simulink model "ICARO3_orientation_controllo_BIPE"  (R2014a)
settings: Solver=FixedStepDiscrete  SolverMode=MultiTasking  StartTime=0.0  StopTime=inf  FixedStep=0.001  RelTol=1e-3
PreLoadFcn:
  | Icaro_path;
  | 
  | load_param;
  | 
  | %override compute_alloc_inside load_param !!!
  | compute_alloc_esa;
  | 
  | load('mag_calib_sim_HIL.mat');
  | 
  | init_adaptive;
InitFcn:
  | %define fast control loop sample time
  | ST = 0.005;
  | 
  | %define filters
  | s = tf('s');
  | 
  | % Derivator (useful in PID controller)
  | D = 0.01*s/(0.01*s+1);
  | 
  | % LP 2nd order filter
  | LP = 42.88/(3.5*s^2 + 19.6*s + 42.88);
  | 
  | %load new DP position controllers
  | progetto_controllo_pos_v1;
undefined symbols (not defined in the file): DiscIntNeverNeededParam, Earth, G, H, INV_PITCH_RANGE, INV_ROLL_RANGE, INV_THROTTLE_RANGE, INV_YAW_RANGE, PITCH_IDX, PITCH_MID, ROLL_IDX, ROLL_MID, RTOL, THROTTLE_DOWN, THROTTLE_IDX, THROTTLE_LOW_THRES, Ts, WGS84, YAW_IDX, YAW_MID
libraries: simulink x15, GPIO_Lib x3, cstblocks x2, aerolibtransform2 x1, STM32_Config_Lib x1
(part 3 of 5)

== system ICARO3_orientation_controllo_BIPE/debug telemtry FLIGHT TEST/GPS ==
  note: lat lon alt_gps gps_status alt_baro_raw
  note: gps: lat, lon, msl_alt, fix_mode + 100*data_valid
  Mux2 : Mux  Inputs=2
  Mux7 : Mux  Inputs=2
  Rate Transition1 : RateTransition  Deterministic=off
  Rate Transition14 : RateTransition  Deterministic=off
  Selector1 : Selector  IndexMode=Zero-based  InputPortWidth=10  Indices=[2]
  Selector2 : Selector  InputPortWidth=2  Indices=2
  Selector3 : Selector  IndexMode=Zero-based  InputPortWidth=10  Indices=[0 1 8]
  Sum : Sum  Inputs=++|
  detect if was 1 in the last 10 samples : Subsystem
  offset : Gain  Gain=100
  GPS : Outport
  wires:
  [TH] -> Selector2/1
  Rate Transition14/1 -> Mux7/2
  [GPS_data] -> Selector3/1, Selector1/1
  Rate Transition1/1 -> Mux7/1
  [GPS_flag] -> detect if was 1 in the last 10 samples/1(In)
  Mux2/1 -> Rate Transition1/1
  Selector3/1 -> Mux2/1
  Selector1/1 -> Sum/2
  Sum/1 -> Mux2/2
  offset/1 -> Sum/1
  Selector2/1 -> Rate Transition14/1
  Mux7/1 -> GPS/1
  detect if was 1 in the last 10 samples/1(Out) -> offset/1

== system ICARO3_orientation_controllo_BIPE/debug telemtry FLIGHT TEST/GPS ECEF ==
  note: CAMBIAMENTI:
      | - Il presente subsystem
      | - wrap_gpsparser
      | - sfun_gpsparser
      | - Latch di ECEF_ref al primo fix GPS
  Demux : Demux  Outputs=[3 3 ]
  Product : Product  Multiplication=Matrix(*)  RndMeth=Zero
  Product1 : Product  Multiplication=Matrix(*)  RndMeth=Zero
  Rate Transition : RateTransition  OutPortSampleTime=1/100
  Rate Transition1 : RateTransition  OutPortSampleTime=1/100
  Sum : Sum  Inputs=-+|
  NED_p : Outport
  NED_v : Outport  Port=2
  wires:
  [ECEF2NED] -> Rate Transition/1
  [ECEF_ref] -> Rate Transition1/1
  Product/1 -> NED_p/1
  Product1/1 -> NED_v/1
  [GPS_data_ECEF] -> Demux/1
  Demux/1 -> Sum/2
  Rate Transition1/1 -> Sum/1
  Sum/1 -> Product/2
  Rate Transition/1 -> Product/1, Product1/1
  Demux/2 -> Product1/2

== system ICARO3_orientation_controllo_BIPE/debug telemtry FLIGHT TEST/MODIFIED Raw IMU data MPU only + RPY AHRS + ALTITUDE (H Hd 0) to be used for AHRS online tuning ==
  ext input : Inport
  Constant : Constant  Value=0  SampleTime=ST
  Manual Switch1 : ManualSwitch  CurrentSetting=0
  Manual Switch2 : ManualSwitch  CurrentSetting=0
  Manual Switch3 : ManualSwitch  CurrentSetting=0
  Mux1 : Mux  Inputs=[3 2 1]
  Mux12 : Mux
  raw imu data : Outport
  wires:
  [MAG_HMC] -> Mux12/4
  Mux1/1 -> Mux12/1
  [RPY_AHRS] -> Mux1/1
  Mux12/1 -> raw imu data/1  "raw_imu_data"
  [H_HD] -> Mux1/2
  Manual Switch3/1 -> Mux12/2
  Manual Switch1/1 -> Mux12/3
  [GYRO_MPU] -> Manual Switch3/2
  [GYRO_ADIS] -> Manual Switch3/1
  [ACC_MPU] -> Manual Switch1/2
  [ACC_ADIS] -> Manual Switch1/1
  Manual Switch2/1 -> Mux1/3
  Constant/1 -> Manual Switch2/1
  ext input/1 -> Manual Switch2/2

== system ICARO3_orientation_controllo_BIPE/debug telemtry FLIGHT TEST/Raw IMU data MPU + HMC + ADC ==
  Mux12 : Mux
  get 1 2 3 4 6 8 : Selector  InputPortWidth=12  Indices=[1 2 3 4 6 8]
  raw imu data : Outport
  wires:
  get 1 2 3 4 6 8/1 -> Mux12/1
  [MAG_HMC] -> Mux12/4
  [ACC_MPU] -> Mux12/3
  [GYRO_MPU] -> Mux12/2
  Mux12/1 -> raw imu data/1  "raw_imu_data"
  [RC_all_channels_usec] -> get 1 2 3 4 6 8/1

== system ICARO3_orientation_controllo_BIPE/debug telemtry FLIGHT TEST/Raw IMU data MPU only + ADC ==
  Mux1 : Mux  Inputs=6
  Mux12 : Mux
  Rate Transition1 : RateTransition  Deterministic=off  OutPortSampleTime=ST
  raw imu data : Outport
  wires:
  Mux12/1 -> raw imu data/1  "raw_imu_data"
  [I_batt] -> Mux1/2
  [V_batt] -> Mux1/1
  [V_batt_filt] -> Mux1/3
  [I_batt_filt] -> Mux1/4
  [P_batt_filt] -> Mux1/5
  [I_consumption_Ah] -> Mux1/6
  Mux1/1 -> Rate Transition1/1
  [GYRO_MPU] -> Mux12/2
  [ACC_MPU] -> Mux12/3
  [MAG_HMC] -> Mux12/4
  Rate Transition1/1 -> Mux12/1

== system ICARO3_orientation_controllo_BIPE/debug telemtry FLIGHT TEST/Raw IMU data packer ==
  Mux12 : Mux  Inputs=5
  raw imu data : Outport
  wires:
  [ACC_MPU] -> Mux12/1
  [GYRO_MPU] -> Mux12/2
  [MAG_HMC] -> Mux12/5
  [GYRO_ITG] -> Mux12/3
  [ACC_ADXL] -> Mux12/4
  Mux12/1 -> raw imu data/1  "raw_imu_data"

== system ICARO3_orientation_controllo_BIPE/debug telemtry FLIGHT TEST/To be used for ADAPT NN online tuning ==
  Mux12 : Mux  Inputs=5
  Selector1 : Selector  InputPortWidth=12  Indices=[7 8 9]
  Selector2 : Selector  InputPortWidth=12  Indices=[10 11 12]
  Selector3 : Selector  InputPortWidth=12  Indices=[1 2 3]
  Selector4 : Selector  InputPortWidth=12  Indices=[4 5 6]
  DEBUG_adapt_contr : Outport
  wires:
  [RPY_AHRS] -> Mux12/1
  Mux12/1 -> DEBUG_adapt_contr/1
  [debug_ADAPT_CONTR] -> Selector2/1, Selector1/1, Selector4/1, Selector3/1
  Selector3/1 -> Mux12/2
  Selector4/1 -> Mux12/3
  Selector1/1 -> Mux12/4
  Selector2/1 -> Mux12/5

== system ICARO3_orientation_controllo_BIPE/debug telemtry FLIGHT TEST/To be used for H PID online tuning ==
  note: hb, zd, 0
  note: y_ref, y, 0
  note: H pid -> D, P, I
  ext input : Inport
  Constant : Constant  Value=0  SampleTime=ST
  Constant1 : Constant  Value=0  SampleTime=ST
  Constant2 : Constant  Value=0  SampleTime=ST
  Manual Switch2 : ManualSwitch  CurrentSetting=0
  Mux1 : Mux  Inputs=[3 2 1]
  Mux12 : Mux
  Mux2 : Mux  Inputs=2
  Mux3 : Mux  Inputs=2
  Selector1 : Selector  InputPortWidth=5  Indices=[1 2 3]
  Selector2 : Selector  InputPortWidth=5  Indices=[4 5]
  raw imu data : Outport
  wires:
  ext input/1 -> Manual Switch2/2
  Constant/1 -> Manual Switch2/1
  Manual Switch2/1 -> Mux1/3
  [H_HD] -> Mux1/2
  Mux12/1 -> raw imu data/1  "raw_imu_data"
  [RPY_AHRS] -> Mux1/1
  Mux1/1 -> Mux12/1
  [debug_H_PID] -> Selector2/1, Selector1/1
  Selector1/1 -> Mux12/2
  Selector2/1 -> Mux3/1
  Constant2/1 -> Mux3/2
  Mux3/1 -> Mux12/3
  [filtInput_debugHPID] -> Mux2/1
  Constant1/1 -> Mux2/2
  Mux2/1 -> Mux12/4

== system ICARO3_orientation_controllo_BIPE/debug telemtry FLIGHT TEST/recupero di mpu9150 data ==
  Mux1 : Mux  Inputs=2
  raw imu data : Outport
  wires:
  Mux1/1 -> raw imu data/1
  [ACC_MPU] -> Mux1/1
  [GYRO_MPU] -> Mux1/2

== system ICARO3_orientation_controllo_BIPE/debug telemtry FLIGHT TEST/test solo RC_all_channel_usec + RSSI + .... ==
  Mux12 : Mux
  Rate Transition1 : RateTransition  Deterministic=off  OutPortSampleTime=ST
  Rate Transition2 : RateTransition  Deterministic=off  OutPortSampleTime=ST
  get 1 2 3 4 6 8 : Selector  InputPortWidth=12  Indices=[1 2 3 4 6 8]
  raw imu data : Outport
  wires:
  get 1 2 3 4 6 8/1 -> Rate Transition1/1
  [RC_all_channels_usec] -> get 1 2 3 4 6 8/1
  Mux12/1 -> raw imu data/1  "raw_imu_data"
  Rate Transition1/1 -> Mux12/1
  [RSSI_VOLT] -> Rate Transition2/1
  [RC_TRPY_refs] -> Mux12/3
  [RC_age] -> Mux12/4
  Rate Transition2/1 -> Mux12/2

== system ICARO3_orientation_controllo_BIPE/debug telemtry FLIGHT TEST1/MODIFIED Raw IMU data MPU only + RPY AHRS + ALTITUDE (H Hd 0) to be used for AHRS online tuning ==
  Mux12 : Mux
  raw imu data : Outport
  wires:
  Mux12/1 -> raw imu data/1  "raw_imu_data"
  [RPY_AHRS_AR] -> Mux12/1
  [ACC_MPU] -> Mux12/2
  [GYRO_MPU] -> Mux12/3
  [H_HD] -> Mux12/4

== system ICARO3_orientation_controllo_BIPE/debug telemtry STATIC TEST/Raw IMU data packer: MPU + MAG_HMC ==
  Manual Switch8 : ManualSwitch  CurrentSetting=0
  Mux12 : Mux  Inputs=3
  raw imu data : Outport
  wires:
  Mux12/1 -> raw imu data/1  "raw_imu_data"
  [GYRO_MPU] -> Mux12/1
  [ACC_MPU] -> Mux12/2
  Manual Switch8/1 -> Mux12/3
  [MAG_MPU] -> Manual Switch8/1
  [MAG_HMC] -> Manual Switch8/2

== system ICARO3_orientation_controllo_BIPE/debug telemtry STATIC TEST/Subsystem ==
  Mux12 : Mux  Inputs=2
  debias_imu_mpu : Outport
  wires:
  [gyro_det_mpu] -> Mux12/2
  Mux12/1 -> debias_imu_mpu/1
  [acc_det_mpu] -> Mux12/1

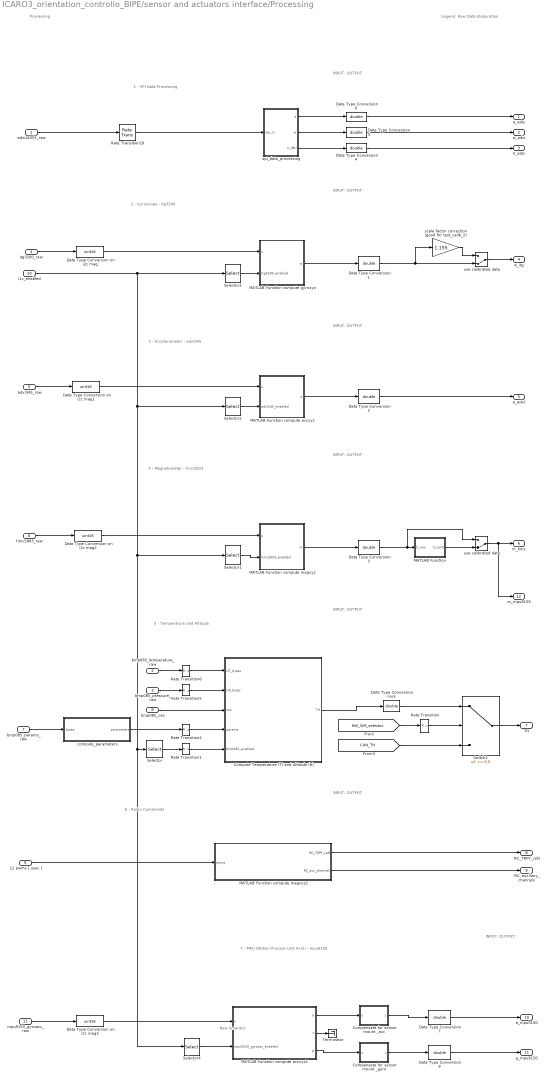
== system ICARO3_orientation_controllo_BIPE/sensor and actuators interface/Processing ==
  note: New Smarabr
  note: Processing
  note: 2 - Gyroscope - itg3200
  note: 1 - SPI Data Processing
  note: 3 - Accelerometer - adxl345
  note: 4 - Magnetometer - hmc5833
  note: 7 - MPU (Motion Process Unit A+G) - mpu9150
  note: 5 - Temperature and Altitude
  note: 6 - Radio Commands
  note: Legend: Raw Data Elaboration
  note: INPUT:
      |
      | OUTPUT:
  note: INPUT:
      |
      | OUTPUT:
  note: INPUT:
      |
      | OUTPUT:
  note: INPUT:
      |
      | OUTPUT:
  note: INPUT:
      |
      | OUTPUT:
  note: INPUT:
      |
      | OUTPUT:
  note: INPUT:
      |
      | OUTPUT:
  adis16355_raw : Inport
  bmp085_temperature_raw : Inport  Port=2
  bmp085_pressure_raw : Inport  Port=3
  itg3200_raw : Inport  Port=4
  adxl345_raw : Inport  Port=5
  hmc5883_raw : Inport  Port=6
  bmp085_params_raw : Inport  Port=7
  bmp085_oss : Inport  Port=8
  12 pwms [ usec ] : Inport  Port=9
  i2c_enabled : Inport  Port=10
  mpu9150_gyroacc_raw : Inport  Port=11
  Compensate for sensor mount _acc : MATLAB Function  TreatAsAtomicUnit=on
  Compensate for sensor mount _gyro : MATLAB Function  TreatAsAtomicUnit=on
  Compute Temperature (T) and Altitude (H) : Subsystem  TreatAsAtomicUnit=on  SystemSampleTime=0.02
  Data Type Conversion mx5 : DataTypeConversion  OutDataTypeStr=double  RndMeth=Round  SaturateOnIntegerOverflow=on
  Data Type Conversion on i2c mag{,1..3} (4 alike) : DataTypeConversion  OutDataTypeStr=uint16
  Data Type Conversion{1..7,9} (8 alike) : DataTypeConversion  OutDataTypeStr=double
  MATLAB Function : MATLAB Function  TreatAsAtomicUnit=on
  MATLAB Function compute accxyz : MATLAB Function  TreatAsAtomicUnit=on
  MATLAB Function compute accxyz1 : MATLAB Function  TreatAsAtomicUnit=on
  MATLAB Function compute gyroxyz : MATLAB Function  TreatAsAtomicUnit=on
  MATLAB Function compute magxyz : MATLAB Function  TreatAsAtomicUnit=on
  MATLAB Function compute magxyz2 : MATLAB Function  TreatAsAtomicUnit=on
  Rate Transition : RateTransition
  Rate Transition{1..2,5..6,18} (5 alike) : RateTransition  Deterministic=off
  Selector : Selector  InputPortWidth=6  Indices=5
  Selector1 : Selector  InputPortWidth=6  Indices=[4]
  Selector2 : Selector  InputPortWidth=6  Indices=3
  Selector3 : Selector  InputPortWidth=6  Indices=[2]
  Selector4 : Selector  InputPortWidth=6  Indices=6
  Switch2 : Switch  Threshold=0.5
  Terminator : Terminator
  compute_parameters : Subsystem
  scale factor correction (good for test_calib_2) : Gain  Gain=1.155
  spi_data_processing : Subsystem
  use calibrated data : ManualSwitch  CurrentSetting=0
  "use calibrated data " : ManualSwitch  CurrentSetting=0
  a_adis : Outport
  w_adis : Outport  Port=2
  V_adis : Outport  Port=3
  w_itg : Outport  Port=4
  a_adxl : Outport  Port=5
  m_hmc : Outport  Port=6
  TH : Outport  Port=7
  RC_TRPY_refs : Outport  Port=8
  RC_auxiliary_channels : Outport  Port=9
  a_mpu9150 : Outport  Port=10
  g_mpu9150 : Outport  Port=11
  m_mpu9150 : Outport  Port=12
  wires:
  Selector4/1 -> MATLAB Function compute accxyz1/2(mpu9150_gyroacc_enabled)
  Data Type Conversion on i2c mag3/1 -> MATLAB Function compute accxyz1/1(u)
  MATLAB Function compute accxyz1/3(g) -> Compensate for sensor mount _gyro/1(u)
  MATLAB Function compute accxyz1/2(t) -> Terminator/1
  Data Type Conversion9/1 -> g_mpu9150/1
  Data Type Conversion7/1 -> a_mpu9150/1
  mpu9150_gyroacc_raw/1 -> Data Type Conversion on i2c mag3/1
  bmp085_temperature_raw/1 -> Rate Transition6/1
  bmp085_pressure_raw/1 -> Rate Transition5/1
  Rate Transition2/1 -> Compute Temperature (T) and Altitude (H)/4(params)
  Rate Transition1/1 -> Compute Temperature (T) and Altitude (H)/5(bmp085_enabled)
  MATLAB Function compute magxyz/1(m) -> Data Type Conversion3/1
  MATLAB Function compute accxyz/1(a) -> Data Type Conversion2/1
  MATLAB Function compute gyroxyz/1(w) -> Data Type Conversion1/1
  Selector/1 -> Rate Transition1/1
  compute_parameters/1(parameters) -> Rate Transition2/1
  Rate Transition/1 -> Switch2/2
  [HW_SIM_selector] -> Rate Transition/1
  [CAN_TH] -> Switch2/3
  Data Type Conversion mx5/1 -> Switch2/1
  Switch2/1 -> TH/1
  scale factor correction (good for test_calib_2)/1 -> "use calibrated data "/1
  "use calibrated data "/1 -> w_itg/1
  use calibrated data/1 -> m_hmc/1, m_mpu9150/1
  MATLAB Function/1(h_calib) -> use calibrated data/2
  Selector3/1 -> MATLAB Function compute gyroxyz/2(itg3200_enabled)
  Selector2/1 -> MATLAB Function compute accxyz/2(adxl345_enabled)
  Selector1/1 -> MATLAB Function compute magxyz/2(hmc5833_enabled)
  i2c_enabled/1 -> Selector1/1, Selector4/1, Selector/1, Selector2/1, Selector3/1
  12 pwms [ usec ]/1 -> MATLAB Function compute magxyz2/1(pwms)
  Data Type Conversion6/1 -> a_adis/1
  Data Type Conversion5/1 -> w_adis/1
  Data Type Conversion4/1 -> V_adis/1
  bmp085_params_raw/1 -> compute_parameters/1(bytes)
  hmc5883_raw/1 -> Data Type Conversion on i2c mag2/1
  adxl345_raw/1 -> Data Type Conversion on i2c mag1/1
  itg3200_raw/1 -> Data Type Conversion on i2c mag/1
  spi_data_processing/3(V_IMU) -> Data Type Conversion4/1
  spi_data_processing/2(w) -> Data Type Conversion5/1
  adis16355_raw/1 -> Rate Transition18/1
  spi_data_processing/1(a) -> Data Type Conversion6/1
  Compute Temperature (T) and Altitude (H)/1(TH) -> Data Type Conversion mx5/1
  Data Type Conversion on i2c mag/1 -> MATLAB Function compute gyroxyz/1(u)
  Data Type Conversion on i2c mag1/1 -> MATLAB Function compute accxyz/1(u)
  Data Type Conversion on i2c mag2/1 -> MATLAB Function compute magxyz/1(u)
  Rate Transition18/1 -> spi_data_processing/1(spi_rx)
  bmp085_oss/1 -> Compute Temperature (T) and Altitude (H)/3(oss)
  Rate Transition6/1 -> Compute Temperature (T) and Altitude (H)/1(UT_bytes)
  Rate Transition5/1 -> Compute Temperature (T) and Altitude (H)/2(UP_bytes)
  MATLAB Function compute magxyz2/1(RC_TRPY_refs) -> RC_TRPY_refs/1
  MATLAB Function compute magxyz2/2(RC_aux_channels) -> RC_auxiliary_channels/1
  Data Type Conversion1/1 -> scale factor correction (good for test_calib_2)/1, "use calibrated data "/2
  Data Type Conversion2/1 -> a_adxl/1
  Data Type Conversion3/1 -> use calibrated data/1, MATLAB Function/1(h_raw)
  MATLAB Function compute accxyz1/1(a) -> Compensate for sensor mount _acc/1(u)
  Compensate for sensor mount _acc/1(y) -> Data Type Conversion7/1
  Compensate for sensor mount _gyro/1(y) -> Data Type Conversion9/1

== matlab function ICARO3_orientation_controllo_BIPE/debug telemtry FLIGHT TEST/MATLAB Function2 ==
  settings: updateMethod=DISCRETE  sampleTime=ST
  data: in input; out output
function out  = findmax(in)
%#codegen

persistent m;

if(isempty(m))
    m = 0;
end

if (in > m)
    m = in;
end

out = m;

== matlab function ICARO3_orientation_controllo_BIPE/debug telemtry FLIGHT TEST/join enable flags ==
  data: u input; y output uint8
function y = join_enable_flags(u)
%#codegen

%compress i2c enable flags into bits:
%MSB [motors press gyro acc mag gyroacc_mpu mag_mpu 0] LSB
%
%from wrap_i2c_requests.c:
%     output[22 + MOTORS_IDX]          = i2c_enabled[MOTORS_IDX];
%     output[22 + PRESS_IDX]           = i2c_enabled[PRESS_IDX];
%     output[22 + GYRO_IDX]            = i2c_enabled[GYRO_IDX];
%     output[22 + ACC_IDX]             = i2c_enabled[ACC_IDX];
%     output[22 + MAG_IDX]             = i2c_enabled[MAG_IDX];
%     output[22 + MPU9150_GYROACC_IDX] = i2c_enabled[MPU9150_GYROACC_IDX];
%     output[22 + MPU9150_MAG_IDX]     = i2c_enabled[MPU9150_MAG_IDX];
y = u(1)*128+u(2)*64+u(3)*32+u(4)*16+u(5)*8+u(6)*4;%+u(7)*2;

== matlab function ICARO3_orientation_controllo_BIPE/debug telemtry STATIC TEST/join enable flags ==
  data: u input; y output uint8
function y = join_enable_flags(u)
%#codegen

%compress i2c enable flags into bits:
%MSB [motors press gyro acc mag 0 0 0 ] LSB
%
%from wrap_i2c_requests.c:
%     output[22 + MOTORS_IDX] = i2c_enabled[MOTORS_IDX];
%     output[22 + PRESS_IDX] = i2c_enabled[PRESS_IDX];
%     output[22 + GYRO_IDX] = i2c_enabled[GYRO_IDX];
%     output[22 + ACC_IDX] = i2c_enabled[ACC_IDX];
%     output[22 + MAG_IDX] = i2c_enabled[MAG_IDX];
%     output[22 + MPU9150_GYROACC_IDX] = i2c_enabled[MPU9150_GYROACC_IDX];
%     output[22 + MPU9150_MAG_IDX] = i2c_enabled[MPU9150_MAG_IDX];
y = u(1)*128+u(2)*64+u(3)*32+u(4)*16+u(5)*8+u(6)*4; %+u(7)*2;

== matlab function ICARO3_orientation_controllo_BIPE/sensor and actuators interface/interrupt manager/CANbus data RX/Subsystem3/MATLAB Function compute gyroxyz1 ==
  settings: updateMethod=DISCRETE  sampleTime=0.01
  data: u input uint16; y output uint16
function y   = pack2_16bit(u)

y = bitor(bitshift(u(2), 8),u(1));

end

== matlab function ICARO3_orientation_controllo_BIPE/sensor and actuators interface/interrupt manager/CANbus data RX/Subsystem3/MATLAB Function compute gyroxyz2 ==
  settings: updateMethod=DISCRETE  sampleTime=0.01
  data: u input uint16; y output uint16
function y   = pack2_16bit(u)

y = bitor(bitshift(u(2), 8),u(1));

end

== matlab function ICARO3_orientation_controllo_BIPE/sensor and actuators interface/interrupt manager/CANbus data RX/Subsystem3/MATLAB Function compute gyroxyz3 ==
  settings: updateMethod=DISCRETE  sampleTime=0.01
  data: u input uint16; y output uint16
function y   = pack2_16bit(u)

y = bitor(bitshift(u(2), 8),u(1));

end

== matlab function ICARO3_orientation_controllo_BIPE/sensor and actuators interface/interrupt manager/CANbus data RX/Subsystem3/MATLAB Function compute gyroxyz5 ==
  settings: updateMethod=DISCRETE  sampleTime=0.01
  data: u input uint16; y output uint16
function y   = pack2_16bit(u)

y = bitor(bitshift(u(2), 8),u(1));

end

== matlab function ICARO3_orientation_controllo_BIPE/sensor and actuators interface/interrupt manager/compose data from canbus/H/typecast uin32 to single ==
  data: u input uint32; y output single
function y = fcn_unit322single(u)
%#codegen

y = typecast(u,'single');

== matlab function ICARO3_orientation_controllo_BIPE/sensor and actuators interface/interrupt manager/compose data from canbus/typecast uin32 to single ==
  data: u input uint32; y output single
function y = fcn_unit322single(u)
%#codegen

y = typecast(u,'single');

== matlab function ICARO3_orientation_controllo_BIPE/sensor and actuators interface/interrupt manager/compose data from canbus/typecast uin32 to single1 ==
  data: u input uint32; y output single
function y = fcn_unit322single(u)
%#codegen

y = typecast(u,'single');

== matlab function ICARO3_orientation_controllo_BIPE/sensor and actuators interface/interrupt manager/send motor commands via canbus/Subsystem10/MATLAB Function compute gyroxyz2 ==
  settings: updateMethod=DISCRETE  sampleTime=0.01
  data: u input uint16; y output uint8
function y = pack2_8bit(u)

y =uint8([0,0]);
y(1) = bitand(u,255);
y(2) = bitshift(u,-8);

== matlab function ICARO3_orientation_controllo_BIPE/sensor and actuators interface/interrupt manager/send motor commands via canbus/Subsystem10/MATLAB Function compute gyroxyz5 ==
  settings: updateMethod=DISCRETE  sampleTime=0.01
  data: u input uint16; y output uint8
function y = pack2_8bit(u)

y =uint8([0,0]);
y(1) = bitand(u,255);
y(2) = bitshift(u,-8);

== matlab function ICARO3_orientation_controllo_BIPE/sensor and actuators interface/interrupt manager/send motor commands via canbus/Subsystem7/MATLAB Function compute gyroxyz3 ==
  settings: updateMethod=DISCRETE  sampleTime=0.01
  data: u input uint16; y output uint8
function y = pack2_8bit(u)

y =uint8([0,0]);
y(1) = bitand(u,255);
y(2) = bitshift(u,-8);

== matlab function ICARO3_orientation_controllo_BIPE/sensor and actuators interface/interrupt manager/send motor commands via canbus/Subsystem8/MATLAB Function compute gyroxyz2 ==
  settings: updateMethod=DISCRETE  sampleTime=0.01
  data: u input uint16; y output uint8
function y = pack2_8bit(u)

y =uint8([0,0]);
y(1) = bitand(u,255);
y(2) = bitshift(u,-8);

== matlab function ICARO3_orientation_controllo_BIPE/Compensate for sensor mount _acc ==
  data: u input; y output
function y = rotX(u)



R=[1 0 0;0 -1 0;0 0 -1];

y =R*u;
end

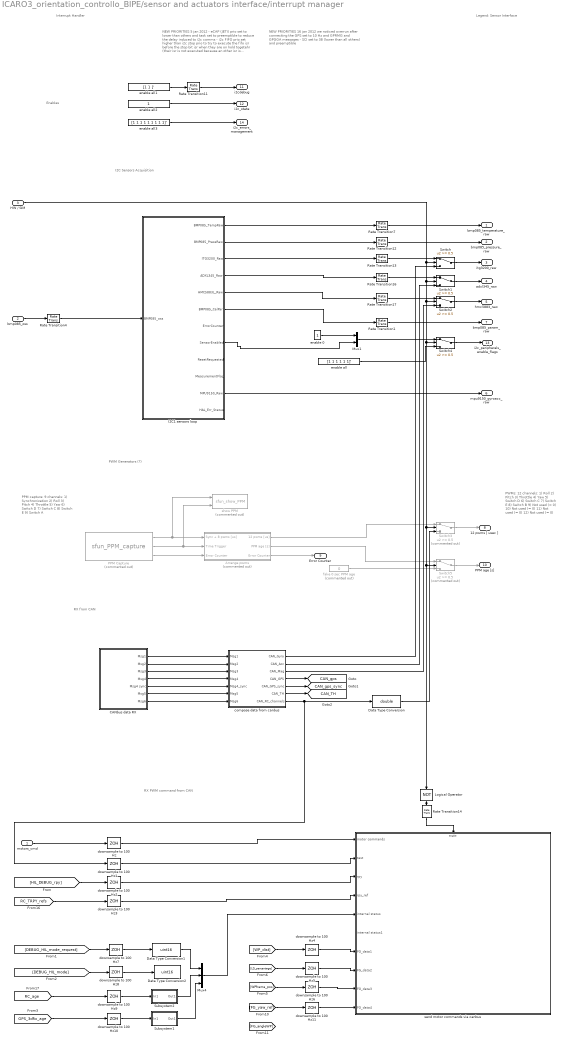
== system ICARO3_orientation_controllo_BIPE/sensor and actuators interface/interrupt manager ==
  note: PWMs: 12 channels:
      |
      | 1) Roll
      | 2) Pitch
      | 3) Throttle
      | 4) Yaw
      | 5) Switch D
      | 6) Switch C
      | 7) Switch E
      | 8) Switch B
      | 9) Not used (= 0)
      | 10) Not used (= 0)
      | 11) Not used (= 0)
      | 12) Not used (= 0)
  note: NEW PRIORITIES
      | 16 jan 2012
      |
      | we noticed overrun after connecting the GPS
      | set to 10 Hz and GPRMG and GPGGA messages
      |
      | - SCI set to 38 (lower than all others)
      |   and preemptible
  note: NEW PRIORITIES
      | 5 jan 2012
      |
      | - eCAP (JETI) prio set to lower than others
      | and task set to preemptible to reduce
      | the delay induced to i2c comms
      |
      | - i2c FIFO prio set higher than i2c stop prio
      | to try to execute the fifo isr before the stop bit isr
      | when they are on hold togetehr (their isr is
      | not executed because an other isr is executing)
  note: PPM capture:
      | 9 channels:
      |
      | 1) Synchronization
      | 2) Roll
      | 3) Pitch
      | 4) Throttle
      | 5) Yaw
      | 6) Switch D
      | 7) Switch C
      | 8) Switch E
      | 9) Switch A
  note: Interrupt Handler
  note: RX PWM command from CAN
  note: Enables
  note: I2C Sensors Acquisition
  note: PWM Generators (?)
  note: RX from CAN
  note: Legend: Sensor Interface
  motors_cmd : Inport
  bmp085_oss : Inport  Port=2
  HW / SIM : Inport  Port=3
  Arrange pwms : Subsystem  Commented=on
  CANbus data RX : Subsystem  TreatAsAtomicUnit=on
  Data Type Conversion : DataTypeConversion  OutDataTypeStr=double
  Data Type Conversion1 : DataTypeConversion  OutDataTypeStr=uint16
  Data Type Conversion2 : DataTypeConversion  OutDataTypeStr=uint16
  I2C1 sensors loop : Subsystem
  Logical Operator : Logic  Operator=NOT  AllPortsSameDT=off  OutDataTypeStr=boolean
  Mux1 : Mux  Inputs=2
  Mux4 : Mux  Inputs=3
  PPM Capture : S-Function  Commented=on  FunctionName=sfun_PPM_capture  Parameters=ST  EnableBusSupport=off
  Rate Transition{1,7,12..13,16..17} (6 alike) : RateTransition  Deterministic=off  OutPortSampleTime=ST
  Rate Transition11 : RateTransition  Deterministic=off
  Rate Transition14 : RateTransition  Deterministic=off
  Rate Transition4 : RateTransition  Deterministic=off
  Subsystem1 : Subsystem
  Subsystem2 : Subsystem
  Switch{,1..2,4} (4 alike) : Switch  Threshold=0.5
  Switch3 : Switch  Commented=on  Threshold=0.5
  Switch5 : Switch  Commented=on  Threshold=0.5
  compose data from canbus : Subsystem
  downsample to 100 Hz{,1..11} (12 alike) : ZeroOrderHold  SampleTime=0.01
  enable 0 : Constant  OutDataTypeStr=uint8
  enable all : Constant  Value=[1 1 1 1 1 1]'  OutDataTypeStr=uint8
  enable all1 : Constant  Value=[1 1 ]'  OutDataTypeStr=uint8
  enable all2 : Constant  OutDataTypeStr=uint8
  enable all3 : Constant  Value=[1 1 1 1 1 1 1 1 1]'  OutDataTypeStr=uint8  SampleTime=ST
  fake 0 sec PPM age : Constant  Commented=on  Value=0
  send motor commands via canbus : Subsystem
  show PPM : S-Function  Commented=on  FunctionName=sfun_show_PPM  Parameters=ST  EnableBusSupport=off
  bmp085_temperature_raw : Outport
  bmp085_pressure_raw : Outport  Port=2
  itg3200_raw : Outport  Port=3
  adxl345_raw : Outport  Port=4
  hmc5883_raw : Outport  Port=5
  mpu9150_gyroacc_raw : Outport  Port=6
  bmp085_param_raw : Outport  Port=7
  12 pwms [ usec ] : Outport  Port=8
  Error Counter : Outport  Port=9
  PPM age [s] : Outport  Port=10
  i2cdebug : Outport  Port=11
  i2c_state : Outport  Port=12
  i2c_peripherals_enable_flags : Outport  Port=13
  i2c_errors_management : Outport  Port=14
  tag scope: CAN_TH=global, CAN_gps=global, CAN_gps_sync=global
  wires:
  I2C1 sensors loop/11(MPU9150_Raw) -> mpu9150_gyroacc_raw/1
  I2C1 sensors loop/8(SensorEnabled) -> Mux1/2
  Mux1/1 -> Switch4/1
  enable 0/1 -> Mux1/1
  Switch4/1 -> i2c_peripherals_enable_flags/1
  enable all/1 -> Switch4/3
  PPM Capture/1 -> Arrange pwms/1(Sync + 8 pwms [us]), show PPM/1
  PPM Capture/2 -> Arrange pwms/2(Time Trigger), show PPM/2
  Arrange pwms/3(Error Counter) -> Error Counter/1
  Arrange pwms/2(PPM age [s]) -> Switch5/1
  Arrange pwms/1(12 pwms [us]) -> Switch3/1
  PPM Capture/3 -> Arrange pwms/3("Error Counter ")
  compose data from canbus/7(CAN_RC_channels) -> downsample to 100 Hz1/1, Data Type Conversion/1
  Rate Transition14/1 -> send motor commands via canbus/Enable
  Rate Transition1/1 -> bmp085_param_raw/1
  enable all3/1 -> i2c_errors_management/1
  enable all2/1 -> i2c_state/1
  I2C1 sensors loop/6(BMP085_CalPar) -> Rate Transition1/1
  downsample to 100 Hz11/1 -> send motor commands via canbus/10(FG_data4)
  [FG_yaw_ref] -> downsample to 100 Hz11/1
  [WPframe_pos] -> downsample to 100 Hz6/1
  [LD_percentage] -> downsample to 100 Hz5/1
  [WP_dist] -> downsample to 100 Hz4/1
  Subsystem1/1(Out1) -> Mux4/3
  Subsystem2/1(Out1) -> Mux4/2
  Data Type Conversion1/1 -> Mux4/1
  downsample to 100 Hz10/1 -> Subsystem1/1(In1)
  [GPS_3dfix_age] -> downsample to 100 Hz10/1
  downsample to 100 Hz9/1 -> Subsystem2/1(In1)
  [RC_age] -> downsample to 100 Hz9/1
  downsample to 100 Hz8/1 -> Data Type Conversion2/1
  [DEBUG_HIL_mode] -> downsample to 100 Hz8/1
  downsample to 100 Hz7/1 -> Data Type Conversion1/1
  [DEBUG_HIL_mode_request] -> downsample to 100 Hz7/1
  Mux4/1 -> send motor commands via canbus/5(internal status)
  downsample to 100 Hz/1 -> send motor commands via canbus/1(motor commands)
  downsample to 100 Hz6/1 -> send motor commands via canbus/9(FG_data3)
  downsample to 100 Hz5/1 -> send motor commands via canbus/8(FG_data2)
  downsample to 100 Hz4/1 -> send motor commands via canbus/7(FG_data1)
  downsample to 100 Hz3/1 -> send motor commands via canbus/4(rpy_ref)
  downsample to 100 Hz2/1 -> send motor commands via canbus/3(rpy)
  [RC_TRPY_refs] -> downsample to 100 Hz3/1
  [HIL_DEBUG_rpy] -> downsample to 100 Hz2/1
  downsample to 100 Hz1/1 -> send motor commands via canbus/2(test)
  Switch5/1 -> PPM age [s]/1
  fake 0 sec PPM age/1 -> Switch5/3
  Logical Operator/1 -> Rate Transition14/1
  Data Type Conversion/1 -> Switch3/3
  compose data from canbus/6(CAN_TH) -> [CAN_TH]
  Switch3/1 -> 12 pwms [ usec ]/1
  compose data from canbus/5(CAN_GPS_sync) -> [CAN_gps_sync]
  compose data from canbus/4(CAN_GPS) -> [CAN_gps]
  Rate Transition17/1 -> Switch2/1
  Rate Transition16/1 -> Switch1/1
  Rate Transition13/1 -> Switch/1
  compose data from canbus/3(CAN_Mag) -> Switch2/3
  compose data from canbus/2(CAN_Acc) -> Switch1/3
  compose data from canbus/1(CAN_Gyro) -> Switch/3
  Switch2/1 -> hmc5883_raw/1
  Switch1/1 -> adxl345_raw/1
  Switch/1 -> itg3200_raw/1
  CANbus data RX/5(Msg4 sync) -> compose data from canbus/5(Msg4_sync)
  CANbus data RX/7(Msg6) -> compose data from canbus/7(Msg6)
  CANbus data RX/6(Msg5) -> compose data from canbus/6(Msg5)
  CANbus data RX/4(Msg4) -> compose data from canbus/4(Msg4)
  CANbus data RX/3(Msg3) -> compose data from canbus/3(Msg3)
  CANbus data RX/2(Msg2) -> compose data from canbus/2(Msg2)
  CANbus data RX/1(Msg1) -> compose data from canbus/1(Msg1)
  HW / SIM/1 -> Logical Operator/1, Switch5/2, Switch3/2, Switch4/2, Switch2/2, Switch1/2, Switch/2
  Rate Transition11/1 -> i2cdebug/1
  enable all1/1 -> Rate Transition11/1
  bmp085_oss/1 -> Rate Transition4/1
  Rate Transition4/1 -> I2C1 sensors loop/1(BMP085_oss)
  motors_cmd/1 -> downsample to 100 Hz/1
  Rate Transition12/1 -> bmp085_pressure_raw/1
  Rate Transition7/1 -> bmp085_temperature_raw/1
  I2C1 sensors loop/5(HMC5883L_Raw) -> Rate Transition17/1
  I2C1 sensors loop/4(ADXL345_Raw) -> Rate Transition16/1
  I2C1 sensors loop/3(ITG3200_Raw) -> Rate Transition13/1
  I2C1 sensors loop/2(BMP085_PressRaw) -> Rate Transition12/1
  I2C1 sensors loop/1(BMP085_TempRaw) -> Rate Transition7/1

== system ICARO3_orientation_controllo_BIPE/ADIS AHRS2/Attitude Filter ADIS/DCM_MARG_QUAT ==
  gyro : Inport
  acc : Inport  Port=2
  mag : Inport  Port=3
  Add3 : Sum  Inputs=+-
  Data Type Conversion mx3 : DataTypeConversion  OutDataTypeStr=single  RndMeth=Round  SaturateOnIntegerOverflow=on
  Discrete-Time Integrator3 : DiscreteIntegrator  SampleTime=T  ICPrevOutput=DiscIntNeverNeededParam  ICPrevScaledInput=DiscIntNeverNeededParam
  Gain1 : Gain  Gain=1/tau
  Scope6 : Scope
      settings: YMin=-0.05  YMax=0.75  SaveName=ScopeData17
  Unit Delay1 : UnitDelay  InitialCondition=[1;0;0;0]  SampleTime=T
  Unit Delay2 : UnitDelay  SampleTime=T
  Unit Delay3 : UnitDelay  SampleTime=T
  dcm_marg : MATLAB Function  TreatAsAtomicUnit=on
  roll_pitch_yaw : Outport
  biases : Outport  Port=2
  a_ned : Outport  Port=3
  q : Outport  Port=4
  wires:
  dcm_marg/6(biases) -> Add3/1
  Unit Delay2/1 -> dcm_marg/5(e_int_a)
  dcm_marg/4(e_int_out_a) -> Unit Delay2/1
  Unit Delay1/1 -> dcm_marg/4(q)
  dcm_marg/3(q_out) -> Unit Delay1/1, q/1
  mag/1 -> dcm_marg/3(mag)
  gyro/1 -> dcm_marg/1(gyro)
  dcm_marg/1(euler_out) -> roll_pitch_yaw/1
  Add3/1 -> Gain1/1
  Gain1/1 -> Discrete-Time Integrator3/1
  Discrete-Time Integrator3/1 -> Add3/2, biases/1
  dcm_marg/2(a_ned) -> a_ned/1
  dcm_marg/5(e_int_out_m) -> Unit Delay3/1
  Unit Delay3/1 -> dcm_marg/6(e_int_m)
  acc/1 -> Data Type Conversion mx3/1
  Data Type Conversion mx3/1 -> dcm_marg/2(acc)
  dcm_marg/7(e_m) -> Scope6/1

== system ICARO3_orientation_controllo_BIPE/ADIS AHRS2/debias ADIS/Acceleration Detrend  ==
  In : Inport
  Detrending : Inport  Port=2
  Demux : Demux  Outputs=3
  Detrend : Subsystem  mask{ST=ST2}
      mask prompts: ST "Sample Time"
  Detrend1 : Subsystem  mask{ST=ST2}
      mask prompts: ST "Sample Time"
  Detrend3 : Subsystem  mask{ST=ST2}
      mask prompts: ST "Sample Time"
  Mux : Mux  Inputs=3
  Out : Outport
  wires:
  Detrend/1(Detrended Output) -> Mux/1
  Detrend1/1(Detrended Output) -> Mux/2
  Detrend3/1(Detrended Output) -> Mux/3
  Mux/1 -> Out/1
  Demux/1 -> Detrend/1(Input)
  Demux/2 -> Detrend1/1(Input)
  In/1 -> Demux/1
  Demux/3 -> Detrend3/1(Input)
  Detrending/1 -> Detrend3/2(Detrending), Detrend/2(Detrending), Detrend1/2(Detrending)

== system ICARO3_orientation_controllo_BIPE/ADIS AHRS2/debias ADIS/Gyros Detrend ==
  In : Inport
  Detrending : Inport  Port=2
  Demux : Demux  Outputs=3
  Detrend : Subsystem  mask{ST=ST2}
      mask prompts: ST "Sample Time"
  Detrend1 : Subsystem  mask{ST=ST2}
      mask prompts: ST "Sample Time"
  Detrend2 : Subsystem  mask{ST=ST2}
      mask prompts: ST "Sample Time"
  Mux : Mux  Inputs=3
  Out : Outport
  wires:
  Detrending/1 -> Detrend2/2(Detrending), Detrend1/2(Detrending), Detrend/2(Detrending)
  Demux/3 -> Detrend2/1(Input)
  In/1 -> Demux/1
  Demux/2 -> Detrend1/1(Input)
  Demux/1 -> Detrend/1(Input)
  Mux/1 -> Out/1
  Detrend2/1(Detrended Output) -> Mux/3
  Detrend1/1(Detrended Output) -> Mux/2
  Detrend/1(Detrended Output) -> Mux/1

== system ICARO3_orientation_controllo_BIPE/ADIS AHRS2/debias ADIS1/Acceleration Detrend  ==
  In : Inport  OutDataTypeStr=single
  Detrending : Inport  Port=2
  Demux : Demux  Outputs=3
  Detrend : Subsystem  mask{ST=ST2}
      mask prompts: ST "Sample Time"
  Detrend1 : Subsystem  mask{ST=ST2}
      mask prompts: ST "Sample Time"
  Detrend3 : Subsystem  mask{ST=ST2}
      mask prompts: ST "Sample Time"
  Mux : Mux  Inputs=3
  Out : Outport
  wires:
  Detrend/1(Detrended Output) -> Mux/1
  Detrend1/1(Detrended Output) -> Mux/2
  Detrend3/1(Detrended Output) -> Mux/3
  Mux/1 -> Out/1
  Demux/1 -> Detrend/1(Input)
  Demux/2 -> Detrend1/1(Input)
  In/1 -> Demux/1
  Demux/3 -> Detrend3/1(Input)
  Detrending/1 -> Detrend3/2(Detrending), Detrend1/2(Detrending), Detrend/2(Detrending)

== system ICARO3_orientation_controllo_BIPE/ADIS AHRS2/debias ADIS1/Acceleration Detrend 1 ==
  In : Inport
  Detrending : Inport  Port=2
  Demux : Demux  Outputs=3
  Detrend : Subsystem  mask{ST=ST2}
      mask prompts: ST "Sample Time"
  Detrend1 : Subsystem  mask{ST=ST2}
      mask prompts: ST "Sample Time"
  Detrend3 : Subsystem  mask{ST=ST2}
      mask prompts: ST "Sample Time"
  Mux : Mux  Inputs=3
  Out : Outport
  wires:
  Detrend/1(Detrended Output) -> Mux/1
  Detrend1/1(Detrended Output) -> Mux/2
  Detrend3/1(Detrended Output) -> Mux/3
  Mux/1 -> Out/1
  Demux/1 -> Detrend/1(Input)
  Demux/2 -> Detrend1/1(Input)
  In/1 -> Demux/1
  Demux/3 -> Detrend3/1(Input)
  Detrending/1 -> Detrend3/2(Detrending), Detrend1/2(Detrending), Detrend/2(Detrending)

== system ICARO3_orientation_controllo_BIPE/ADIS AHRS2/debias ADIS1/Gyros Detrend ==
  In : Inport
  Detrending : Inport  Port=2
  Data Type Conversion mx3 : DataTypeConversion  OutDataTypeStr=double  RndMeth=Round  SaturateOnIntegerOverflow=on
  Demux : Demux  Outputs=3
  Detrend : Subsystem  mask{ST=ST2}
      mask prompts: ST "Sample Time"
  Detrend1 : Subsystem  mask{ST=ST2}
      mask prompts: ST "Sample Time"
  Detrend2 : Subsystem  mask{ST=ST2}
      mask prompts: ST "Sample Time"
  Mux : Mux  Inputs=3
  Out : Outport
  wires:
  Detrending/1 -> Data Type Conversion mx3/1
  Demux/3 -> Detrend2/1(Input)
  In/1 -> Demux/1
  Demux/2 -> Detrend1/1(Input)
  Demux/1 -> Detrend/1(Input)
  Mux/1 -> Out/1
  Detrend2/1(Detrended Output) -> Mux/3
  Detrend1/1(Detrended Output) -> Mux/2
  Detrend/1(Detrended Output) -> Mux/1
  Data Type Conversion mx3/1 -> Detrend2/2(Detrending), Detrend1/2(Detrending), Detrend/2(Detrending)

== system ICARO3_orientation_controllo_BIPE/GPS receiver/compute 3d age/clock latch ==
  note: NOTE: in initial output of outport set to -1000
      | to esnure age is at least 1000 on startup !!!!
  In : Inport
  Enable : EnablePort
  Out : Outport  InitialOutput=-1000
  wires:
  In/1 -> Out/1

== system ICARO3_orientation_controllo_BIPE/GPS receiver/compute age/clock latch ==
  In : Inport
  Enable : EnablePort
  Out : Outport  InitialOutput=-1000
  wires:
  In/1 -> Out/1

== system ICARO3_orientation_controllo_BIPE/SS AHRS/Attitude Filter SS/DCM_MARG_QUAT ==
  gyro : Inport
  acc : Inport  Port=2
  mag : Inport  Port=3
  Add3 : Sum  Inputs=+-
  Discrete-Time Integrator3 : DiscreteIntegrator  SampleTime=T  ICPrevOutput=DiscIntNeverNeededParam  ICPrevScaledInput=DiscIntNeverNeededParam
  Gain1 : Gain  Gain=1/tau
  Unit Delay1 : UnitDelay  InitialCondition=[1;0;0;0]  SampleTime=T
  Unit Delay2 : UnitDelay  SampleTime=T
  Unit Delay3 : UnitDelay  SampleTime=T
  dcm_marg : MATLAB Function  TreatAsAtomicUnit=on
  roll_pitch_yaw : Outport
  biases : Outport  Port=2
  a_ned : Outport  Port=3
  q : Outport  Port=4
  wires:
  Unit Delay3/1 -> dcm_marg/6(e_int_m)
  dcm_marg/5(e_int_out_m) -> Unit Delay3/1
  dcm_marg/2(a_ned) -> a_ned/1
  Discrete-Time Integrator3/1 -> biases/1, Add3/2
  Gain1/1 -> Discrete-Time Integrator3/1
  Add3/1 -> Gain1/1
  dcm_marg/1(euler_out) -> roll_pitch_yaw/1
  gyro/1 -> dcm_marg/1(gyro)
  acc/1 -> dcm_marg/2(acc)
  mag/1 -> dcm_marg/3(mag)
  dcm_marg/3(q_out) -> q/1, Unit Delay1/1
  Unit Delay1/1 -> dcm_marg/4(q)
  dcm_marg/4(e_int_out_a) -> Unit Delay2/1
  Unit Delay2/1 -> dcm_marg/5(e_int_a)
  dcm_marg/6(biases) -> Add3/1

== system ICARO3_orientation_controllo_BIPE/SS AHRS/debias SS/Acceleration Detrend  ==
  In : Inport
  Detrending : Inport  Port=2
  Demux : Demux  Outputs=3
  Detrend : Subsystem  mask{ST=ST2}
      mask prompts: ST "Sample Time"
  Detrend1 : Subsystem  mask{ST=ST2}
      mask prompts: ST "Sample Time"
  Detrend3 : Subsystem  mask{ST=ST2}
      mask prompts: ST "Sample Time"
  Mux : Mux  Inputs=3
  Out : Outport
  wires:
  Detrending/1 -> Detrend1/2(Detrending), Detrend/2(Detrending), Detrend3/2(Detrending)
  Demux/3 -> Detrend3/1(Input)
  In/1 -> Demux/1
  Demux/2 -> Detrend1/1(Input)
  Demux/1 -> Detrend/1(Input)
  Mux/1 -> Out/1
  Detrend3/1(Detrended Output) -> Mux/3
  Detrend1/1(Detrended Output) -> Mux/2
  Detrend/1(Detrended Output) -> Mux/1

== system ICARO3_orientation_controllo_BIPE/SS AHRS/debias SS/Gyros Detrend ==
  In : Inport
  Detrending : Inport  Port=2
  Demux : Demux  Outputs=3
  Detrend : Subsystem  mask{ST=ST2}
      mask prompts: ST "Sample Time"
  Detrend1 : Subsystem  mask{ST=ST2}
      mask prompts: ST "Sample Time"
  Detrend2 : Subsystem  mask{ST=ST2}
      mask prompts: ST "Sample Time"
  Mux : Mux  Inputs=3
  Out : Outport
  wires:
  Detrend/1(Detrended Output) -> Mux/1
  Detrend1/1(Detrended Output) -> Mux/2
  Detrend2/1(Detrended Output) -> Mux/3
  Mux/1 -> Out/1
  Demux/1 -> Detrend/1(Input)
  Demux/2 -> Detrend1/1(Input)
  In/1 -> Demux/1
  Demux/3 -> Detrend2/1(Input)
  Detrending/1 -> Detrend/2(Detrending), Detrend1/2(Detrending), Detrend2/2(Detrending)

== system ICARO3_orientation_controllo_BIPE/configurazione relativa seeker//target/engagement/Fading filter del II ordine ==
  sigma : Inport
  G1 : Gain  Gain=Ts
  Sum : Sum  Inputs=-+|
  Sum1 : Sum  Inputs=|++
  Sum2 : Sum  Inputs=|++
  Sum3 : Sum  Inputs=+|+
  Unit Delay : UnitDelay  SampleTime=-1
  Unit Delay2 : UnitDelay  SampleTime=-1
  gain : Gain  Gain=G
  gain2 : Gain  Gain=H/Ts
  sigma punto stimata : Outport
  wires:
  Sum/1 -> gain/1, gain2/1
  gain/1 -> Sum1/1
  Sum1/1 -> Unit Delay2/1
  Unit Delay2/1 -> Sum2/2
  Sum2/1 -> Sum1/2, Sum/1
  G1/1 -> Sum2/1
  gain2/1 -> Sum3/1
  Unit Delay/1 -> Sum3/2, G1/1
  Sum3/1 -> Unit Delay/1, sigma punto stimata/1
  sigma/1 -> Sum/2

== system ICARO3_orientation_controllo_BIPE/debug telemtry FLIGHT TEST/GPS/detect if was 1 in the last 10 samples ==
  In : Inport
  Data Type Conversion : DataTypeConversion  OutDataTypeStr=boolean
  Data Type Conversion1 : DataTypeConversion  OutDataTypeStr=double
  Logical Operator3 : Logic  Operator=OR  Inputs=10  AllPortsSameDT=off  OutDataTypeStr=boolean
  Unit Delay{,1..8} (9 alike) : UnitDelay  SampleTime=-1
  Out : Outport
  wires:
  Logical Operator3/1 -> Data Type Conversion1/1
  In/1 -> Data Type Conversion/1
  Unit Delay2/1 -> Logical Operator3/4, Unit Delay3/1
  Unit Delay4/1 -> Logical Operator3/6, Unit Delay5/1
  Unit Delay3/1 -> Logical Operator3/5, Unit Delay4/1
  Unit Delay1/1 -> Logical Operator3/3, Unit Delay2/1
  Unit Delay/1 -> Logical Operator3/2, Unit Delay1/1
  Unit Delay6/1 -> Unit Delay7/1, Logical Operator3/8
  Unit Delay7/1 -> Unit Delay8/1, Logical Operator3/9
  Unit Delay5/1 -> Unit Delay6/1, Logical Operator3/7
  Unit Delay8/1 -> Logical Operator3/10
  Data Type Conversion/1 -> Logical Operator3/1, Unit Delay/1
  Data Type Conversion1/1 -> Out/1

== system ICARO3_orientation_controllo_BIPE/sensor and actuators interface/Processing/Compute Temperature (T) and Altitude (H) ==
  UT_bytes : Inport
  UP_bytes : Inport  Port=2
  oss : Inport  Port=3
  params : Inport  Port=4
  bmp085_enabled : Inport  Port=5
  Data Type Conversion1 : DataTypeConversion  OutDataTypeStr=single
  Data Type Conversion3 : DataTypeConversion  OutDataTypeStr=single
  Data Type Conversion4 : DataTypeConversion  OutDataTypeStr=uint16
  Data Type Conversion5 : DataTypeConversion  OutDataTypeStr=uint32
  Gain1 : Gain  Gain=0.1
  Gain2 : Gain
  MATLAB Function : MATLAB Function  TreatAsAtomicUnit=on
  MATLAB Function1 : MATLAB Function  TreatAsAtomicUnit=on
  Mux : Mux  Inputs=2
  TH : Outport
  wires:
  bmp085_enabled/1 -> MATLAB Function/5(bmp085_enabled)
  Mux/1 -> TH/1
  params/1 -> MATLAB Function/4(params)
  Gain1/1 -> Mux/1
  Gain2/1 -> Mux/2
  MATLAB Function/2(h) -> Gain2/1
  MATLAB Function/1(T) -> Gain1/1
  Data Type Conversion3/1 -> MATLAB Function/2(UP)
  Data Type Conversion1/1 -> MATLAB Function/1(UT)
  Data Type Conversion5/1 -> MATLAB Function1/2(UP_bytes)
  Data Type Conversion4/1 -> MATLAB Function1/1(UT_bytes)
  MATLAB Function1/1(UT) -> Data Type Conversion1/1
  MATLAB Function1/2(UP) -> Data Type Conversion3/1
  oss/1 -> MATLAB Function1/3(oss), MATLAB Function/3(oss)
  UP_bytes/1 -> Data Type Conversion5/1
  UT_bytes/1 -> Data Type Conversion4/1

== system ICARO3_orientation_controllo_BIPE/sensor and actuators interface/Processing/compute_parameters ==
  bytes : Inport
  Data Type Conversion : DataTypeConversion  OutDataTypeStr=uint16
  MATLAB Function1 : MATLAB Function  TreatAsAtomicUnit=on
  parameters : Outport
  wires:
  Data Type Conversion/1 -> MATLAB Function1/1(bytes)
  MATLAB Function1/1(params) -> parameters/1
  bytes/1 -> Data Type Conversion/1

== system ICARO3_orientation_controllo_BIPE/sensor and actuators interface/Processing/spi_data_processing ==
  spi_rx : Inport
  Bitwise Operator : simulink/Logic and Bit Operations/Bitwise Operator  logicop=AND  UseBitMask=on  BitMask=bin2dec('0000111111111111')  BitMaskRealWorld=Stored Integer
  Bitwise Operator{1..6} (6 alike) : simulink/Logic and Bit Operations/Bitwise Operator  logicop=AND  UseBitMask=on  BitMask=bin2dec('0011111111111111')  BitMaskRealWorld=Stored Integer
  Data Type Conversion mx1 : DataTypeConversion  OutDataTypeStr=double  RndMeth=Round  SaturateOnIntegerOverflow=on
  Demux : Demux  Outputs=7
  Gain : Gain  Gain=1.8315/1000
  MATLAB Function compute magxyz1 : MATLAB Function  TreatAsAtomicUnit=on  SystemSampleTime=ST
  Mux : Mux  Inputs=6
  a : Outport
  w : Outport  Port=2
  V_IMU : Outport  Port=3
  wires:
  Gain/1 -> V_IMU/1
  Data Type Conversion mx1/1 -> Gain/1
  Bitwise Operator/1 -> Data Type Conversion mx1/1
  Bitwise Operator6/1 -> Mux/6
  Bitwise Operator5/1 -> Mux/5
  Bitwise Operator4/1 -> Mux/4
  Bitwise Operator3/1 -> Mux/3
  Bitwise Operator2/1 -> Mux/2
  Bitwise Operator1/1 -> Mux/1
  Demux/7 -> Bitwise Operator6/1
  spi_rx/1 -> Demux/1
  Demux/6 -> Bitwise Operator5/1
  Demux/5 -> Bitwise Operator4/1
  Demux/4 -> Bitwise Operator3/1
  Demux/3 -> Bitwise Operator2/1
  Demux/2 -> Bitwise Operator1/1
  Demux/1 -> Bitwise Operator/1
  MATLAB Function compute magxyz1/2(w) -> w/1
  MATLAB Function compute magxyz1/1(a) -> a/1
  Mux/1 -> MATLAB Function compute magxyz1/1(u)

== system ICARO3_orientation_controllo_BIPE/sensor and actuators interface/interrupt manager/Arrange pwms ==
  Sync + 8 pwms [us] : Inport
  Time Trigger : Inport  Port=2
  "Error Counter " : Inport  Port=3
  Demux : Demux  Outputs=[1 8]
  Digital Clock : DigitalClock  SampleTime=ST
  Expected 12 channel: Filling with zeros : Constant  Value=[0 0 0 0]  OutDataTypeStr=uint32
  Mux1 : Mux  Inputs=2
  Rate Transition2 : RateTransition  Deterministic=off
  Rate Transition8 : RateTransition  Deterministic=off
  Rate Transition9 : RateTransition  Deterministic=off
  Sum : Sum  Inputs=|-+
  Sync : Terminator
  clock latch : Subsystem  TreatAsAtomicUnit=on
  12 pwms [us] : Outport
  PPM age [s] : Outport  Port=2
  Error Counter : Outport  Port=3
  wires:
  Demux/1 -> Sync/1
  Demux/2 -> Mux1/1
  Mux1/1 -> Rate Transition8/1
  Sync + 8 pwms [us]/1 -> Demux/1
  Digital Clock/1 -> clock latch/1(In), Sum/2
  Sum/1 -> PPM age [s]/1
  Expected 12 channel: Filling with zeros/1 -> Mux1/2
  Rate Transition2/1 -> Sum/1
  clock latch/1(Out) -> Rate Transition2/1
  Rate Transition8/1 -> 12 pwms [us]/1
  Rate Transition9/1 -> Error Counter/1
  "Error Counter "/1 -> Rate Transition9/1
  Time Trigger/1 -> clock latch/Enable

== system ICARO3_orientation_controllo_BIPE/sensor and actuators interface/interrupt manager/CANbus data RX ==
  note: Modified parameters from 4*ST to
      | 2*ST because the base rate is now 0.005
  note: NOTE: Msg4, Msg5 and Msg6 MUST be
      |            re-assemblate to form a 32, 16, 16 bit packet
  CANRX : S-Function  FunctionName=sfun_CAN_Receive  Parameters=2*ST,6  EnableBusSupport=off
  Demux1 : Demux  Outputs=[8 8 8 8 8 8]
  Mux : Mux  Inputs=6
  New_Message : Terminator
  Rx_ID1 : Constant  Value=bin2dec('11000001111')  OutDataTypeStr=uint32
  Rx_ID2 : Constant  Value=bin2dec('10000001111')  OutDataTypeStr=uint32
  Rx_ID3 : Constant  Value=bin2dec('01100001111')  OutDataTypeStr=uint32
  Rx_ID4 : Constant  Value=bin2dec('01000001111')  OutDataTypeStr=uint32
  Rx_ID5 : Constant  Value=bin2dec('00100001111')  OutDataTypeStr=uint32
  Rx_ID6 : Constant  Value=bin2dec('11100001111')  OutDataTypeStr=uint32
  Subsystem1 : Subsystem
  Subsystem2 : Subsystem
  Subsystem3 : Subsystem
  Msg1 : Outport
  Msg2 : Outport  Port=2
  Msg3 : Outport  Port=3
  Msg4 : Outport  Port=4
  Msg4 sync : Outport  Port=5
  Msg5 : Outport  Port=6
  Msg6 : Outport  Port=7
  wires:
  CANRX/2 -> New_Message/1
  Subsystem1/1(Out1) -> Msg5/1
  Demux1/5 -> Subsystem1/1(In1)
  Demux1/6 -> Subsystem3/1(In1)
  Subsystem3/1(Out1) -> Msg6/1
  Subsystem2/1(Out1) -> Msg4/1
  Demux1/4 -> Subsystem2/1(In1)
  Mux/1 -> CANRX/1
  Rx_ID6/1 -> Mux/6
  Rx_ID5/1 -> Mux/5
  Rx_ID4/1 -> Mux/4
  Rx_ID3/1 -> Mux/3
  Rx_ID2/1 -> Mux/2
  Rx_ID1/1 -> Mux/1
  CANRX/1 -> Demux1/1
  Demux1/3 -> Msg3/1
  Demux1/2 -> Msg2/1
  Demux1/1 -> Msg1/1

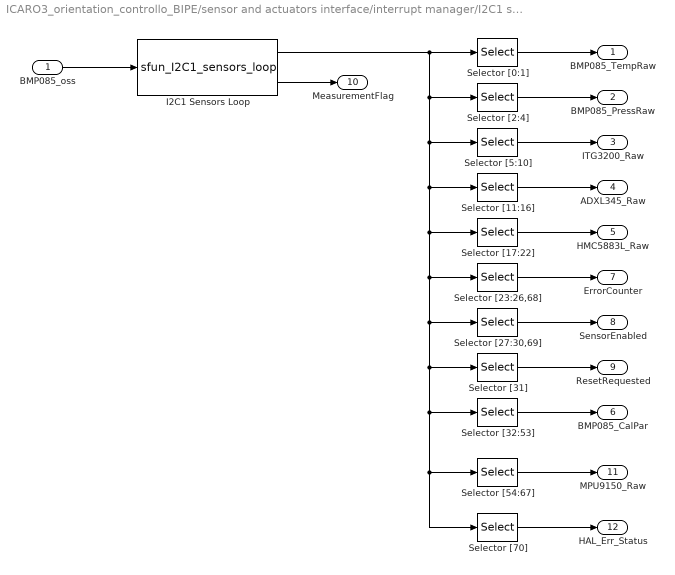
== system ICARO3_orientation_controllo_BIPE/sensor and actuators interface/interrupt manager/I2C1 sensors loop ==
  BMP085_oss : Inport
  I2C1 Sensors Loop : S-Function  FunctionName=sfun_I2C1_sensors_loop  Parameters=ST  EnableBusSupport=off
  Selector [0:1] : Selector  IndexMode=Zero-based  InputPortWidth=71  Indices=[0:1]
  Selector [11:16] : Selector  IndexMode=Zero-based  InputPortWidth=71  Indices=[11:16]
  Selector [17:22] : Selector  IndexMode=Zero-based  InputPortWidth=71  Indices=[17:22]
  Selector [23:26,68] : Selector  IndexMode=Zero-based  InputPortWidth=71  Indices=[23:26,68]
  Selector [27:30,69] : Selector  IndexMode=Zero-based  InputPortWidth=71  Indices=[27:30,69]
  Selector [2:4] : Selector  IndexMode=Zero-based  InputPortWidth=71  Indices=[2:4]
  Selector [31] : Selector  IndexMode=Zero-based  InputPortWidth=71  Indices=[31]
  Selector [32:53] : Selector  IndexMode=Zero-based  InputPortWidth=71  Indices=[32:53]
  "Selector [54:67] " : Selector  IndexMode=Zero-based  InputPortWidth=71  Indices=[54:67]
  Selector [5:10] : Selector  IndexMode=Zero-based  InputPortWidth=71  Indices=[5:10]
  "Selector [70] " : Selector  IndexMode=Zero-based  InputPortWidth=71  Indices=[54:67]
  BMP085_TempRaw : Outport
  BMP085_PressRaw : Outport  Port=2
  ITG3200_Raw : Outport  Port=3
  ADXL345_Raw : Outport  Port=4
  HMC5883L_Raw : Outport  Port=5
  BMP085_CalPar : Outport  Port=6
  ErrorCounter : Outport  Port=7
  SensorEnabled : Outport  Port=8
  ResetRequested : Outport  Port=9
  MeasurementFlag : Outport  Port=10
  MPU9150_Raw : Outport  Port=11
  HAL_Err_Status : Outport  Port=12
  wires:
  "Selector [70] "/1 -> HAL_Err_Status/1
  "Selector [54:67] "/1 -> MPU9150_Raw/1
  Selector [31]/1 -> ResetRequested/1
  Selector [27:30,69]/1 -> SensorEnabled/1
  Selector [23:26,68]/1 -> ErrorCounter/1
  Selector [32:53]/1 -> BMP085_CalPar/1
  Selector [17:22]/1 -> HMC5883L_Raw/1
  Selector [11:16]/1 -> ADXL345_Raw/1
  Selector [2:4]/1 -> BMP085_PressRaw/1
  Selector [5:10]/1 -> ITG3200_Raw/1
  I2C1 Sensors Loop/2 -> MeasurementFlag/1
  Selector [0:1]/1 -> BMP085_TempRaw/1
  I2C1 Sensors Loop/1 -> Selector [0:1]/1, Selector [31]/1, Selector [32:53]/1, "Selector [54:67] "/1, "Selector [70] "/1, Selector [27:30,69]/1, Selector [23:26,68]/1, Selector [17:22]/1, Selector [11:16]/1, Selector [5:10]/1, Selector [2:4]/1
  BMP085_oss/1 -> I2C1 Sensors Loop/1

== system ICARO3_orientation_controllo_BIPE/sensor and actuators interface/interrupt manager/Subsystem1 ==
  In1 : Inport
  Constant : Constant  Value=2047  SampleTime=0.01
  Data Type Conversion2 : DataTypeConversion  OutDataTypeStr=uint16
  Gain : Gain  Gain=100
  Sum : Sum  Inputs=|++
  Out1 : Outport
  wires:
  In1/1 -> Gain/1
  Data Type Conversion2/1 -> Out1/1
  Sum/1 -> Data Type Conversion2/1
  Constant/1 -> Sum/2
  Gain/1 -> Sum/1

== system ICARO3_orientation_controllo_BIPE/sensor and actuators interface/interrupt manager/Subsystem2 ==
  In1 : Inport
  Constant : Constant  Value=2047  SampleTime=0.01
  Data Type Conversion2 : DataTypeConversion  OutDataTypeStr=uint16
  Gain : Gain  Gain=100
  Sum : Sum  Inputs=|++
  Out1 : Outport
  wires:
  Gain/1 -> Sum/1
  Constant/1 -> Sum/2
  Sum/1 -> Data Type Conversion2/1
  Data Type Conversion2/1 -> Out1/1
  In1/1 -> Gain/1
